simulink model "TP1_simulink"  (R2024a)
settings: Solver=VariableStepAuto  StartTime=0.0  StopTime=10.0  RelTol=1e-3
settings Model: Creator=pedro.campos-afonso-  LastModifiedBy=pedro.campos-afonso-

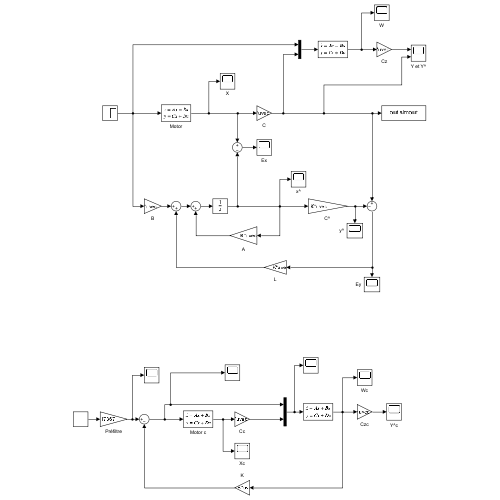
[thumbnail: Simulink's stored preview of the top-level diagram]
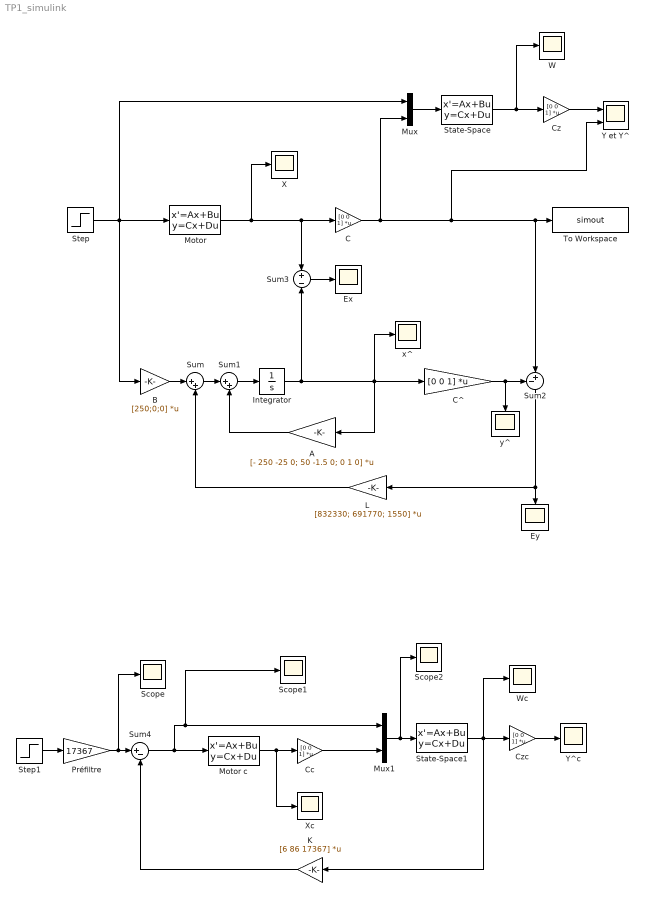
== system TP1_simulink ==
  A : Gain  Gain=[- 250 -25 0; 50 -1.5 0; 0 1 0]  Multiplication=Matrix(K*u) (u vector)
  B : Gain  Gain=[250;0;0]  Multiplication=Matrix(K*u) (u vector)
  C : Gain  Gain=[0 0 1]  Multiplication=Matrix(K*u) (u vector)
  "C^ " : Gain  Gain=[0 0 1]  Multiplication=Matrix(K*u) (u vector)
  Cc : Gain  Gain=[0 0 1]  Multiplication=Matrix(K*u) (u vector)
  Cz : Gain  Gain=[0 0 1]  Multiplication=Matrix(K*u) (u vector)
  Czc : Gain  Gain=[0 0 1]  Multiplication=Matrix(K*u) (u vector)
  Ex : Scope
  Ey : Scope
  Integrator : Integrator
  K : Gain  Gain=[6 86 17367]  Multiplication=Matrix(K*u) (u vector)
  L : Gain  Gain=[832330; 691770; 1550]  Multiplication=Matrix(K*u) (u vector)
  Motor : StateSpace  A=[- 250 -25 0; 50 -1.5 0; 0 1 0]  B=[250;0;0]  C=[1 0 0; 0 1 0; 0 0 1]  D=[0;0;0]  InitialCondition=[0.01;0.02;0.03]
  Motor c : StateSpace  A=[- 250 -25 0; 50 -1.5 0; 0 1 0]  B=[250;0;0]  C=[1 0 0; 0 1 0; 0 0 1]  D=[0;0;0]  InitialCondition=[0.01;0.02;0.03]
  Mux : Mux  Inputs=2
  Mux1 : Mux  Inputs=2
  Préfiltre : Gain  Gain=17367
  Scope : Scope
  Scope1 : Scope
  Scope2 : Scope
  State-Space : StateSpace  A=[-250 -30 -832330; 50 -1.5 -691770; 0 1 -1550]  B=[250 832330; 0 691770; 0 1550]  C=[1 0 0; 0 1 0; 0 0 1]  D=[0 0; 0 0; 0 0]  InitialCondition=0
  State-Space1 : StateSpace  A=[-250 -30 -832330; 50 -1.5 -691770; 0 1 -1550]  B=[250 832330; 0 691770; 0 1550]  C=[1 0 0; 0 1 0; 0 0 1]  D=[0 0; 0 0; 0 0]  InitialCondition=0
  Step : Step  SampleTime=0
  Step1 : Step  SampleTime=0
  Sum : Sum  Inputs=|++
  Sum1 : Sum  Inputs=|++
  Sum2 : Sum  Inputs=-+|
  Sum3 : Sum  Inputs=+|-
  Sum4 : Sum  Inputs=|+-
  To Workspace : ToWorkspace  VariableName=simout  SaveFormat=Timeseries  SampleTime=-1
  W : Scope
  Wc : Scope
  X : Scope
  Xc : Scope
  Y et Y^ : Scope  NumInputPorts=2
  Y^c : Scope
  x^ : Scope
  y^ : Scope
  wires:
  Step/1 -> Mux/1, B/1, Motor/1
  Sum1/1 -> Integrator/1
  "C^ "/1 -> Sum2/1, y^/1
  Motor/1 -> C/1, Sum3/1, X/1
  Sum2/1 -> Ey/1, L/1
  L/1 -> Sum/2
  B/1 -> Sum/1
  Sum/1 -> Sum1/1
  A/1 -> Sum1/2
  Integrator/1 -> A/1, "C^ "/1, x^/1, Sum3/2
  C/1 -> Mux/2, Y et Y^/2, To Workspace/1, Sum2/2
  Sum3/1 -> Ex/1
  Mux/1 -> State-Space/1
  State-Space/1 -> Cz/1, W/1
  Cz/1 -> Y et Y^/1
  Czc/1 -> Y^c/1
  State-Space1/1 -> K/1, Wc/1, Czc/1
  Cc/1 -> Mux1/2
  Motor c/1 -> Xc/1, Cc/1
  Step1/1 -> Préfiltre/1
  Mux1/1 -> Scope2/1, State-Space1/1
  Préfiltre/1 -> Scope/1, Sum4/1
  Sum4/1 -> Scope1/1, Mux1/1, Motor c/1
  K/1 -> Sum4/2
